simulink model "farenheit_to_celsius"  (R2017a)
settings: Solver=VariableStepAuto  StartTime=0.0  StopTime=18  RelTol=1e-3
settings Model: Creator=Priyesh  LastModifiedBy=Priyesh

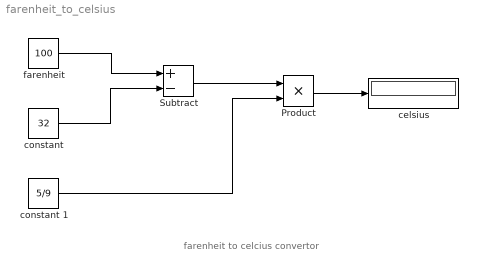
== system farenheit_to_celsius ==
  note: farenheit to celcius convertor
  Product : Product
  Subtract : Sum  Inputs=+-
  "celsius " : Display
  "constant " : Constant  Value=32
  constant 1 : Constant  Value=5/9
  farenheit : Constant  Value=100
  wires:
  farenheit/1 -> Subtract/1
  "constant "/1 -> Subtract/2
  Subtract/1 -> Product/1
  constant 1/1 -> Product/2
  Product/1 -> "celsius "/1
